simulink model "RL_Model"  (R2025b)
settings: Solver=ode14x  StartTime=0  StopTime=100  FixedStep=simStepSize  RelTol=1e-3
undefined symbols (not defined in the file or in its folder): Defined, driving, Ego, Lane, simStepSize, User
libraries: roadrunnerscenario x6, drivingscenarioandsensors x3, simulink_extras x2, rllib x1
settings Model: Creator=Jacob  LastModifiedBy=balls
settings RTWCC: GPUComputeCapability=3.5

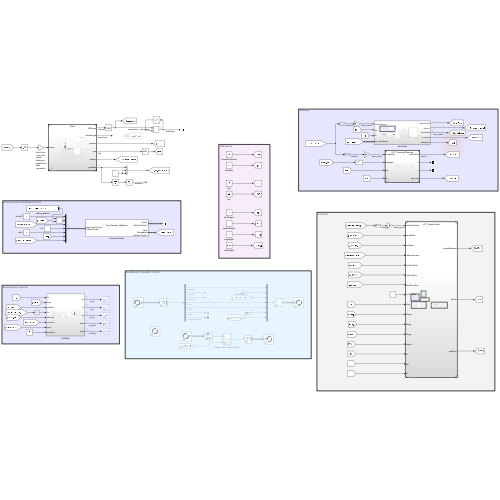
[thumbnail: Simulink's stored preview of the top-level diagram]
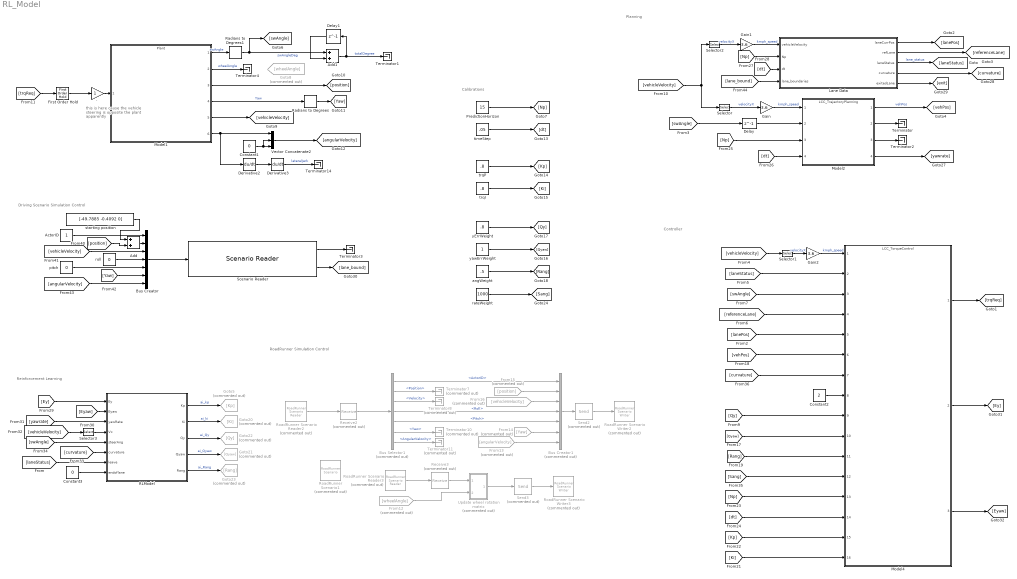
== system RL_Model ==
  note: Driving Scenario Simulation Control
  note: Reinforcement Learning
  note: this is here
      |  cause the
      | vehicle
      | steering is
      | opposite the
      | plant
      |  apparently
  note: Calibrations
  note: Controller
  note: RoadRunner Simulation Control
  note: Planning
  ActorID : Constant
  Add : Sum
  Add1 : Sum
  Bus Creator : BusCreator  Inputs=7  OutDataTypeStr=Bus: BusActorPose  NonVirtualBus=on
      settings: InheritFromInputs=off
  Bus Creator1 : BusCreator  Commented=on  Inputs=7  OutDataTypeStr=Bus: BusActorPose  NonVirtualBus=on
  Bus Selector1 : BusSelector  Commented=on  OutputSignals=ActorID,Position,Velocity,Roll,Pitch,Yaw,AngularVelocity
  Constant1 : Constant  Value=0
  Constant2 : Constant  Value=2
  Constant3 : Constant  Value=0
  Delay : Delay  DelayLength=1
  Delay1 : Delay  DelayLength=1
  Derivative2 : Derivative
  Derivative3 : Derivative
  First Order Hold : FirstOrderHold  ErrorTolerance=inf  AllowContinuousInput=on
  From12 : From  Commented=on  GotoTag=wheelAngle
  From13 : From  Commented=on  GotoTag=angularVelocity
  From14 : From  Commented=on  GotoTag=Yaw
  From15 : From  Commented=on  GotoTag=position
  From16 : From  Commented=on  GotoTag=vehicleVelocity
  Gain : Gain  Gain=3.6
  Gain1 : Gain  Gain=3.6
  Gain2 : Gain  Gain=3.6
  Goto20 : Goto  Commented=on  GotoTag=Ki
  Goto21 : Goto  Commented=on  GotoTag=Qyaw
  Goto22 : Goto  Commented=on  GotoTag=Qy
  Goto23 : Goto  Commented=on  GotoTag=Rang
  Goto5 : Goto  Commented=on  GotoTag=Kp
  Goto8 : Goto  Commented=on  GotoTag=wheelAngle
  Lane Data : Subsystem
  Model1 : ModelReference  ModelNameDialog=Plant.slx  SimulationMode=Normal  ModelReferenceVersion=5.13
  Model2 : ModelReference  ModelNameDialog=LCC_TrajectoryPlanning.slx  SimulationMode=Normal  ModelReferenceVersion=5.4
  Model4 : ModelReference  ModelNameDialog=LCC_TorqueControl.slx  SimulationMode=Normal  ModelReferenceVersion=5.86
  PredictionHorizon : Constant  Value=15
  RLModel : Subsystem
  Radians to Degrees : simulink_extras/Transformations/Radians to Degrees
  Radians to Degrees1 : simulink_extras/Transformations/Radians to Degrees
  Receive2 : Receive  Commented=on  InputPortMessageModes=m  UseInternalQueue=off  QueueOverwriting=on  QueueLength=1  QueueType=LIFO
  Receive3 : Receive  Commented=on  InputPortMessageModes=m  UseInternalQueue=off  QueueOverwriting=on  QueueLength=1  QueueType=LIFO  SampleTime=simStepSize
  RoadRunner Scenario Reader2 : roadrunnerscenario/RoadRunner Scenario Reader  Commented=on  TopicCategory=Actor  ActorCategory=All Types  ActionType=Path Following  EventType=User-Defined  TopicType=Actor Pose (Driving Scenario compatible)  VehicleType=Vehicle Specifications  TrafficSignalType=Traffic Signal Specifications  TrafficSignalControllerType=Traffic Signal Controller Specifications  UserDefinedAction=Action1  UserDefinedEvent=Event1  Filter=Self  AdditionalRelationship=None  SensorTopic=Target Poses  LaneBoundaryOutputTopic=Ego-Lane  SensorID=1  SampleTime=simStepSize
  RoadRunner Scenario Reader3 : roadrunnerscenario/RoadRunner Scenario Reader  Commented=on  TopicCategory=Actor  ActorCategory=Vehicle  ActionType=Path Following  EventType=User-Defined  TopicType=Actor Pose (Driving Scenario compatible)  VehicleType=Vehicle Pose  TrafficSignalType=Traffic Signal Specifications  TrafficSignalControllerType=Traffic Signal Controller Specifications  UserDefinedAction=Action1  UserDefinedEvent=Event1  Filter=Self  AdditionalRelationship=None  SensorTopic=Target Poses  LaneBoundaryOutputTopic=Ego-Lane  SensorID=1  SampleTime=simStepSize
  RoadRunner Scenario Writer2 : roadrunnerscenario/RoadRunner Scenario Writer  Commented=on  TopicCategory=Actor  ActorCategory=All Types  EventType=Action Complete  UserDefinedEvent=Event1  VehicleType=Vehicle Pose  TopicType=Actor Pose (Driving Scenario compatible)
  RoadRunner Scenario Writer3 : roadrunnerscenario/RoadRunner Scenario Writer  Commented=on  TopicCategory=Actor  ActorCategory=Vehicle  EventType=Action Complete  UserDefinedEvent=Event1  VehicleType=Vehicle Pose  TopicType=Actor Pose (Driving Scenario compatible)
  RoadRunner Scenario1 : roadrunnerscenario/RoadRunner Scenario  Commented=on  UserDefinedActions={}  UserDefinedEvents={}  PathPoints=500
  Scenario Reader : drivingscenarioandsensors/Scenario Reader  ScenarioSource=From file  ScenarioFileName=C:\Users\balls\Desktop\EcoCAR\git\CAV - 2025b\Test_Scenario_RightCurv.mat  ScenarioVariableName=scenario  OutputCoordinateSystem=Vehicle coordinates  EgoVehicleSource=Input port  EgoVehicleActorID=1  OrientVehiclesOnRoad=off  OutputEgoVehiclePose=off  OutputEgoVehicleState=off  SampleTime=simStepSize  LaneBoundaryOutput=Ego vehicle lane boundaries  LaneBoundaryDistance=linspace(-150, 150, 101)  LaneBoundaryLocation=Center of lane markings  BusNameSource=Auto  BusName=BusActors  BusNumActorsSource=Scenario  BusNumActors=100  BusName2Source=Auto  BusName2=BusLaneBoundaries  BusNumLaneBoundariesSource=Scenario  BusNumLaneBoundaries=10  BusName3Source=Auto  BusName3=BusEgoActor  BusName4Source=Auto  BusName4=BusEgoState  ShowCoordinateLabels=on  SimulateUsing=Interpreted execution
  Selector{,1..3} (4 alike) : Selector  InputPortWidth=3  IndexOptions=Index vector (dialog)  Indices=1  OutputSizes=1
  Send2 : Send  Commented=on  OutputPortMessageModes=m
  Send3 : Send  Commented=on  OutputPortMessageModes=m
  Terminator{,1..4,14} (6 alike) : Terminator
  Terminator{7..8,10..11} (4 alike) : Terminator  Commented=on
  Update wheel rotation matrix : Subsystem  Commented=on
  Vector Concatenate2 : Concatenate  NumInputs=3  Mode=Multidimensional array  ConcatenateDimension=2
  ` : Gain
  angWeight : Constant  Value=.5
  pitch : Constant  Value=0
  rateWeight : Constant  Value=1000
  roll : Constant  Value=0
  starting position : Constant  Value=[-49.7885 -0.4092 0]
  timeStep : Constant  Value=.05
  trqI : Constant  Value=.8
  trqP : Constant  Value=.8
  yErrWeight : Constant  Value=.8
  yawErrWeight : Constant
  wires:
  Delay1/1 -> Add1/2
  Radians to Degrees1/1 -> [swAngle], Add1/1  "swAngleDeg"
  Bus Selector1/4 -> Bus Creator1/4  "<Roll>"
  From14/1 -> Bus Creator1/6
  Add1/1 -> Terminator1/1, Delay1/1  "totalDegree"
  Bus Selector1/2 -> Terminator7/1  "<Position>"
  Bus Selector1/7 -> Terminator11/1  "<AngularVelocity>"
  Model1/3 -> [position]
  Bus Selector1/1 -> Bus Creator1/1  "<ActorID>"
  RoadRunner Scenario Reader3/1 -> Receive3/1
  Send3/1 -> RoadRunner Scenario Writer3/1
  From15/1 -> Bus Creator1/2
  Model1/4 -> Radians to Degrees/1  "Yaw"
  Derivative2/1 -> Derivative3/1
  Send2/1 -> RoadRunner Scenario Writer2/1
  Model1/1 -> Radians to Degrees1/1  "swAngle"
  Bus Creator1/1 -> Send2/1
  RoadRunner Scenario Reader2/1 -> Receive2/1
  Radians to Degrees/1 -> [Yaw]
  Bus Selector1/5 -> Bus Creator1/5  "<Pitch>"
  Model2/1 -> [vehPos]  "vehPos"
  Receive2/1 -> Bus Selector1/1
  [vehicleVelocity] -> Selector2/1, Selector/1
  Vector Concatenate2/1 -> [angularVelocity]
  Bus Selector1/6 -> Terminator10/1  "<Yaw>"
  Constant1/1 -> Vector Concatenate2/2, Vector Concatenate2/3
  From16/1 -> Bus Creator1/3
  Derivative3/1 -> Terminator14/1  "lateralJerk"
  From13/1 -> Bus Creator1/7
  Model1/5 -> [vehicleVelocity]
  Bus Selector1/3 -> Terminator8/1  "<Velocity>"
  [trqReq] -> First Order Hold/1
  Lane Data/3(laneStatus) -> [laneStatus]  "lane_status"
  Model1/6 -> Derivative2/1, Vector Concatenate2/1
  Selector/1 -> Gain/1  "velocityX"
  Gain/1 -> Model2/1  "kmph_speed"
  Delay/1 -> Model2/2
  First Order Hold/1 -> `/1
  Lane Data/1(laneCurrPos) -> [lanePos]
  [vehicleVelocity] -> Selector1/1
  Selector1/1 -> Gain2/1  "velocityX"
  [swAngle] -> Delay/1
  Receive3/1 -> Update wheel rotation matrix/1(In1)
  Update wheel rotation matrix/1(Out1) -> Send3/1
  From12/1 -> Update wheel rotation matrix/2(Input)
  [vehPos] -> Model4/6
  [Np] -> Model2/3
  [dt] -> Model2/4
  angWeight/1 -> [Rang]
  yawErrWeight/1 -> [Qyaw]
  yErrWeight/1 -> [Qy]
  trqI/1 -> [Ki]
  trqP/1 -> [Kp]
  timeStep/1 -> [dt]
  PredictionHorizon/1 -> [Np]
  [Qy] -> Model4/9
  [Qyaw] -> Model4/10
  [Rang] -> Model4/11
  [Np] -> Model4/13
  [dt] -> Model4/14
  [Np] -> Lane Data/2(Np)
  [dt] -> Lane Data/3(dt)
  Model4/1 -> [trqReq]
  Selector2/1 -> Gain1/1  "velocityX"
  Gain1/1 -> Lane Data/1(vehicleVelocity)  "kmph_speed"
  Lane Data/2(refLane) -> [referenceLane]
  `/1 -> Model1/1
  RLModel/1(Kp) -> Goto5/1  "ai_kp"
  RLModel/2(Ki) -> Goto20/1  "ai_ki"
  RLModel/3(Qy) -> Goto22/1  "ai_Qy"
  RLModel/4(Qyaw) -> Goto21/1  "ai_Qyaw"
  RLModel/5(Rang) -> Goto23/1  "ai_Rang"
  [Ey] -> RLModel/1(Ey)
  [Eyaw] -> RLModel/2(Eyaw)
  [yawrate] -> RLModel/3(yawRate)
  [vehicleVelocity] -> Selector3/1
  Lane Data/4(curvature) -> [curvature]
  [curvature] -> RLModel/6(curvature)
  [swAngle] -> RLModel/5(steerAng)
  rateWeight/1 -> [Sang]
  [Sang] -> Model4/12
  [curvature] -> Model4/7
  Constant2/1 -> Model4/8
  Lane Data/5(exitedLane) -> [exit]
  [laneStatus] -> RLModel/7(leave)
  Model2/4 -> [yawrate]
  Model2/2 -> Terminator/1
  Model2/3 -> Terminator2/1
  Constant3/1 -> RLModel/8(endoflane)
  Selector3/1 -> RLModel/4(Vx)
  Scenario Reader/2 -> [lane_bound]
  Scenario Reader/1 -> Terminator3/1
  [lane_bound] -> Lane Data/4(lane_boundaries)
  Model1/2 -> Terminator4/1  "wheelAngle"
  ActorID/1 -> Bus Creator/1
  [angularVelocity] -> Bus Creator/7
  [vehicleVelocity] -> Bus Creator/3
  pitch/1 -> Bus Creator/5
  roll/1 -> Bus Creator/4
  [Yaw] -> Bus Creator/6
  Bus Creator/1 -> Scenario Reader/1
  [position] -> Add/2
  starting position/1 -> Add/1
  Add/1 -> Bus Creator/2
  [Kp] -> Model4/15
  [Ki] -> Model4/16
  [lanePos] -> Model4/5
  [referenceLane] -> Model4/4
  Gain2/1 -> Model4/1  "kmph_speed"
  [swAngle] -> Model4/3
  [laneStatus] -> Model4/2
  Model4/2 -> [Ey]
  Model4/3 -> [Eyaw]

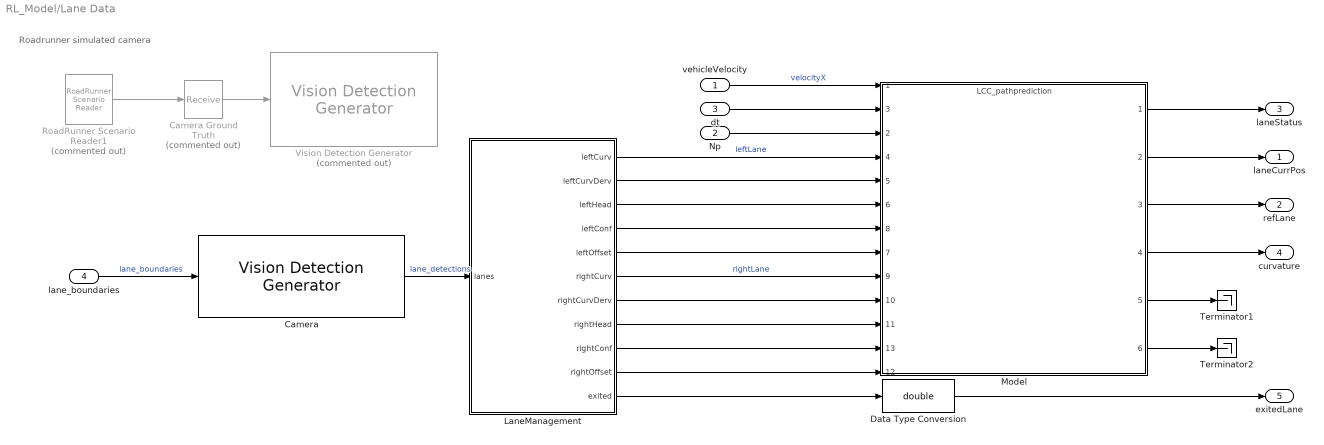
== system RL_Model/Lane Data ==
  note: Roadrunner simulated camera
  vehicleVelocity : Inport
  Np : Inport  Port=2
  dt : Inport  Port=3
  lane_boundaries : Inport  Port=4
  Camera : drivingscenarioandsensors/Vision Detection Generator  SensorIndex=1  DetectorOutput=Lanes only  UpdateInterval=0.1  LaneUpdateInterval=0.1  SensorLocation=[1.9 0]  Height=1.1  Yaw=0  Pitch=1  Roll=0  BusNameSource=Auto  BusName=BusObjectDetections  BusName2Source=Auto  BusName2=BusLaneDetections  MaxNumDetectionsSource=Property  MaxNumDetections=50  MaxNumLanesSource=Property  MaxNumLanes=30  DetectionCoordinates=Ego Cartesian  SimulateUsing=Interpreted execution  MaxRange=150  BoundingBoxAccuracy=5  ProcessNoiseIntensity=5  MaxSpeed=100  MaxAllowedOcclusion=0.5  MinObjectImageSize=[15 15]  DetectionProbability=0.9  FalsePositivesPerImage=0.1  MinLaneImageSize=[20 3]  LaneBoundaryAccuracy=3  HasNoise=on  InitialSeedSource=Repeatable  InitialSeed=0  UsedSeed=0  ActorProfilesSource=From Scenario Reader block  ActorProfilesParameters=driving.internal.ActorProfilesParameters  ActorProfilesExpression=[struct('ActorID',1,'ClassID',1,'Length',4.7,'Width',1.8,'Height',1.4,'OriginOffset',[-1.35 0 0],'MeshVertices',[3.7 0.9 0.857439446366782;3.7 -0.9 0.857439446366782;3.7 -0.9 0.314878892733564;3.7 0.9 0.314878892733564;3.7 0.9 0.857439446366782;2.525 0.9 0.993079584775086;2.525 -0.9 0.993079584775086;3.7 -0.9 0.857439446366782;1.82 0.72 1.4;0.41 0.72 1.4;0.41 -0.72 1.4;1.82 -0.72 1.4;-0.295 0.9 0.993079584775086;-1 0.9 0.857439446366782;-1 -0.9 0.857439446366782;-0.295 -0.9 0.993079584775086;3.7 0.9 0.857439446366782;3.7 0.9 0.314878892733564;2.525 0.9 0.314878892733564;2.525 0.9 0.993079584775086;2.525 0.9 0.993079584775086;2.525 0.9 0.314878892733564;-0.295 0.9 0.314878892733564;-0.295 0.9 0.993079584775086;-0.295 0.9 0.993079584775086;-0.295 0.9 0.314878892733564;-1 0.9 0.355570934256055;-1 0.9 0.857439446366782;2.525 0.9 0.993079584775086;-0.295 0.9 0.993079584775086;0.41 0.72 1.4;1.82 0.72 1.4;3.7 -0.9 0.857439446366782;3.7 -0.9 0.314878892733564;2.525 -0.9 0.314878892733564;2.525 -0.9 0.993079584775086;2.525 -0.9 0.993079584775086;2.525 -0.9 0.314878892733564;-0.295 -0.9 0.314878892733564;-0.295 -0.9 0.993079584775086;-0.295 -0.9 0.993079584775086;-0.295 -0.9 0.314878892733564;-1 -0.9 0.355570934256055;-1 -0.9 0.857439446366782;2.525 -0.9 0.993079584775086;-0.295 -0.9 0.993079584775086;0.41 -0.72 1.4;1.82 -0.72 1.4;-0.295 0.9 0.993079584775086;-0.295 -0.9 0.993079584775086;0.41 -0.72 1.4;0.41 0.72 1.4;2.525 -0.9 0.993079584775086;1.82 -0.72 1.4;1.82 0.72 1.4;2.525 0.9 0.993079584775086;-1 0.9 0.857439446366782;-1 0.9 0.355570934256055;-1 -0.9 0.355570934256055;-1 -0.9 0.857439446366782;3.7 0.9 0.314878892733564;3.7 -0.9 0.314878892733564;-0.295 -0.9 0.314878892733564;-0.295 0.9 0.314878892733564;-0.295 0.9 0.314878892733564;-1 0.9 0.355570934256055;-1 -0.9 0.355570934256055;-0.295 -0.9 0.314878892733564;0 -0.63 0;0 -0.87 0;0.191030206995054 -0.63 0.0601365173421445;0.191030206995054 -0.87 0.0601365173421445;0.309093367795925 -0.63 0.217575963708927;0.309093367795925 -0.87 0.217575963708927;0.309093367795925 -0.63 0.412181821758201;0.309093367795925 -0.87 0.412181821758201;0.191030206995054 -0.63 0.569621268124983;0.191030206995054 -0.87 0.569621268124983;0 -0.63 0.629757785467128;0 -0.87 0.629757785467128;-0.191030206995054 -0.63 0.569621268124983;-0.191030206995054 -0.87 0.569621268124983;-0.309093367795925 -0.63 0.412181821758201;-0.309093367795925 -0.87 0.412181821758201;-0.309093367795925 -0.63 0.217575963708927;-0.309093367795925 -0.87 0.217575963708927;-0.191030206995054 -0.63 0.0601365173421445;-0.191030206995054 -0.87 0.0601365173421445;0 -0.63 0;0 -0.87 0;0 -0.63 0;0.191030206995054 -0.63 0.0601365173421445;0.309093367795925 -0.63 0.217575963708927;0.309093367795925 -0.63 0.412181821758201;0.191030206995054 -0.63 0.569621268124983;0 -0.63 0.629757785467128;-0.191030206995054 -0.63 0.569621268124983;-0.309093367795925 -0.63 0.412181821758201;-0.309093367795925 -0.63 0.217575963708927;-0.191030206995054 -0.63 0.0601365173421445;0 -0.87 0;0.191030206995054 -0.87 0.0601365173421445;0.309093367795925 -0.87 0.217575963708927;0.309093367795925 -0.87 0.412181821758201;0.191030206995054 -0.87 0.569621268124983;0 -0.87 0.629757785467128;-0.191030206995054 -0.87 0.569621268124983;-0.309093367795925 -0.87 0.412181821758201;-0.309093367795925 -0.87 0.217575963708927;-0.191030206995054 -0.87 0.0601365173421445;0 0.87 0;0 0.63 0;0.191030206995054 0.87 0.0601365173421445;0.191030206995054 0.63 0.0601365173421445;0.309093367795925 0.87 0.217575963708927;0.309093367795925 0.63 0.217575963708927;0.309093367795925 0.87 0.412181821758201;0.309093367795925 0.63 0.412181821758201;0.191030206995054 0.87 0.569621268124983;0.191030206995054 0.63 0.569621268124983;0 0.87 0.629757785467128;0 0.63 0.629757785467128;-0.191030206995054 0.87 0.569621268124983;-0.191030206995054 0.63 0.569621268124983;-0.309093367795925 0.87 0.412181821758201;-0.309093367795925 0.63 0.412181821758201;-0.309093367795925 0.87 0.217575963708927;-0.309093367795925 0.63 0.217575963708927;-0.191030206995054 0.87 0.0601365173421445;-0.191030206995054 0.63 0.0601365173421445;0 ...(+3718 chars)],'MeshFaces',[1 2 3;3 4 1;5 6 7;7 8 5;9 10 11;11 12 9;13 14 15;15 16 13;17 18 19;19 20 17;21 22 23;23 24 21;25 26 27;27 28 25;29 30 31;31 32 29;33 34 35;35 36 33;37 38 39;39 40 37;41 42 43;43 44 41;45 46 47;47 48 45;49 50 51;51 52 49;53 54 55;55 56 53;57 58 59;59 60 57;61 62 63;63 64 61;65 66 67;67 68 65;69 71 72;72 70 69;71 73 74;74 72 71;73 75 76;76 74 73;75 77 78;78 76 75;77 79 80;80 78 77;79 81 82;82 80 79;81 83 84;84 82 81;83 85 86;86 84 83;85 87 88;88 86 85;87 89 90;90 88 87;91 92 93;91 93 94;91 94 95;91 95 96;91 96 97;91 97 98;91 98 99;91 99 100;101 102 103;101 103 104;101 104 105;101 105 106;101 106 107;101 107 108;101 108 109;101 109 110;111 113 114;114 112 111;113 115 116;116 114 113;115 117 118;118 116 115;117 119 120;120 118 117;119 121 122;122 120 119;121 123 124;124 122 121;123 125 126;126 124 123;125 127 128;128 126 125;127 129 130;130 128 127;129 131 132;132 130 129;133 134 135;133 135 136;133 136 137;133 137 138;133 138 139;133 139 140;133 140 141;133 141 142;143 144 145;143 145 146;143 146 147;143 147 148;143 148 149;143 149 150;143 150 151;143 151 152;153 155 156;156 154 153;155 157 158;158 156 155;157 159 160;160 158 157;159 161 162;162 160 159;161 163 164;164 162 161;163 165 166;166 164 163;165 167 168;168 166 165;167 169 170;170 168 167;169 171 172;172 170 169;171 173 174;174 172 171;175 176 177;175 177 178;175 178 179;175 179 180;175 180 181;175 181 182;175 182 183;175 183 184;185 186 187;185 187 188;185 188 189;185 189 190;185 190 191;185 191 192;185 192 193;185 193 194;195 197 198;198 196 195;197 199 200;200 198 197;199 201 202;202 200 199;201 203 204;204 202 201;203 205 206;206 204 203;205 207 208;208 206 205;207 209 210;210 208 207;209 211 212;212 210 209;211 213 214;214 212 211;213 215 216;216 214 213;217 218 219;217 219 220;217 220 221;217 221 222;217 222 223;217 223 224;217 224 225;217 225 226;227 228 229;227 229 230;227 230 231;227 231 232;227 232 233;227 233 234;227 234 235;227 235 236],'RCSPattern',[10 10;10 10],'RCSAzimuthAngles',[-180 180],'RCSElevationAngles',[-90 90])]  Intrinsics=driving.internal.cameraIntrinsics('FocalLength',[800 800],'PrincipalPoint',[320 240],'ImageSize',[480 640],'RadialDistortion',[0 0],'TangentialDistortion',[0 0],'Skew',0)
  Camera Ground Truth : Receive  Commented=on  InputPortMessageModes=m  UseInternalQueue=off  QueueOverwriting=on  QueueLength=1  QueueType=LIFO  SampleTime=simStepSize
  Data Type Conversion : DataTypeConversion  OutDataTypeStr=double  SaturateOnIntegerOverflow=off  RndMeth=Floor
  LaneManagement : MATLAB Function  TreatAsAtomicUnit=on
  Model : ModelReference  ModelNameDialog=LCC_pathprediction.slx  SimulationMode=Normal  ModelReferenceVersion=5.49
      settings: PortSchema="{\"entries\":[{\"content\":{\"sides\":[{\"content\":{\"connectorIds\":[\"In1\",\"In3\",\"In2\",\"In4\",\"In5\",\"In6\",\"In8\",\"In7\",\"In9\",\"In10\",\"In11\",\"In13\",\"In12\"]},\"type\":\"ConnectorPlacement.EquallySpacedRectSide\",\"uuid\":\"a07f8485-8c73-44ce-93cf-ec5e6f63c5da\"},{\"content\":{\"connectorIds\":[\"Out1\",\"Out2\",\"Out3\",\"Out4\",\"Out5\",\"Out6\"],\"side\":\"RIGHT\"},\"type\":\"ConnectorPlacement.EquallySpacedRectSide\",\"uuid\":\"b69156b0-73a0-4176-8c64-fda440ac3685\"},{\"content\":{\"side\":\"TOP\"},\"type\":\"ConnectorPlacement.EquallySpacedRectSide\",\"uuid\":\"33404bc1-182d-48ae-8070-d21d23a4a197\"}]},\"type\":\"ConnectorPlacement.EquallySpacedConnector\",\"uuid\":\"de203df0-0780-4dcc-b040-a4939f0923fa\"}],\"packageUris\":[\"http://schema.mathworks.com/mf0/Connector/R2020b\"],\"version\":\"1.0\"}"
  RoadRunner Scenario Reader1 : roadrunnerscenario/RoadRunner Scenario Reader  Commented=on  TopicCategory=Sensor  ActorCategory=All Types  ActionType=Path Following  EventType=User-Defined  TopicType=Actor Specifications  VehicleType=Vehicle Specifications  TrafficSignalType=Traffic Signal Specifications  TrafficSignalControllerType=Traffic Signal Controller Specifications  UserDefinedAction=Action1  UserDefinedEvent=Event1  Filter=Self  AdditionalRelationship=None  SensorTopic=Lane Boundaries  LaneBoundaryOutputTopic=Ego and Adjacent Lanes  SensorID=1  SampleTime=simStepSize
  Terminator1 : Terminator
  Terminator2 : Terminator
  Vision Detection Generator : drivingscenarioandsensors/Vision Detection Generator  Commented=on  SensorIndex=1  DetectorOutput=Lanes only  UpdateInterval=simStepSize  LaneUpdateInterval=simStepSize  SensorLocation=[ 1, 0 ]  Height=1.9  Yaw=0  Pitch=1  Roll=0  BusNameSource=Auto  BusName=BusObjectDetections  BusName2Source=Auto  BusName2=BusLaneDetections  MaxNumDetectionsSource=Property  MaxNumDetections=10  MaxNumLanesSource=Property  MaxNumLanes=10  DetectionCoordinates=Ego Cartesian  SimulateUsing=Code generation  MaxRange=100  BoundingBoxAccuracy=5  ProcessNoiseIntensity=5  MaxSpeed=100  MaxAllowedOcclusion=0.5  MinObjectImageSize=[ 5, 5 ]  DetectionProbability=0.99  FalsePositivesPerImage=0.01  MinLaneImageSize=[ 20, 3 ]  LaneBoundaryAccuracy=3  HasNoise=on  InitialSeedSource=Repeatable  InitialSeed=0  UsedSeed=driving.internal.SimulinkUtilities.seedManager(gcb)  ActorProfilesSource=From Scenario Reader block  ActorProfilesParameters=driving.internal.ActorProfilesParameters  ActorProfilesExpression=struct( 'ClassID', 0, 'Length', 4.7, 'Width', 1.8, 'Height', 1.4, 'OriginOffset', [ -1.35, 0, 0 ] )  Intrinsics=driving.internal.cameraIntrinsics
  laneCurrPos : Outport
  refLane : Outport  Port=2
  laneStatus : Outport  Port=3
  curvature : Outport  Port=4
  exitedLane : Outport  Port=5
  wires:
  RoadRunner Scenario Reader1/1 -> Camera Ground Truth/1
  Model/1 -> laneStatus/1
  Model/2 -> laneCurrPos/1
  Model/3 -> refLane/1
  vehicleVelocity/1 -> Model/1  "velocityX"
  Np/1 -> Model/2
  dt/1 -> Model/3
  Model/5 -> Terminator1/1
  Model/4 -> curvature/1
  LaneManagement/1(leftCurv) -> Model/4  "leftLane"
  LaneManagement/2(leftCurvDerv) -> Model/5
  LaneManagement/3(leftHead) -> Model/6
  LaneManagement/4(leftConf) -> Model/8
  LaneManagement/5(leftOffset) -> Model/7
  LaneManagement/6(rightCurv) -> Model/9  "rightLane"
  LaneManagement/10(rightOffset) -> Model/12
  LaneManagement/9(rightConf) -> Model/13
  LaneManagement/8(rightHead) -> Model/11
  LaneManagement/7(rightCurvDerv) -> Model/10
  Data Type Conversion/1 -> exitedLane/1
  LaneManagement/11(exited) -> Data Type Conversion/1
  Camera Ground Truth/1 -> Vision Detection Generator/1
  Camera/1 -> LaneManagement/1(lanes)  "lane_detections"
  lane_boundaries/1 -> Camera/1  "lane_boundaries"
  Model/6 -> Terminator2/1

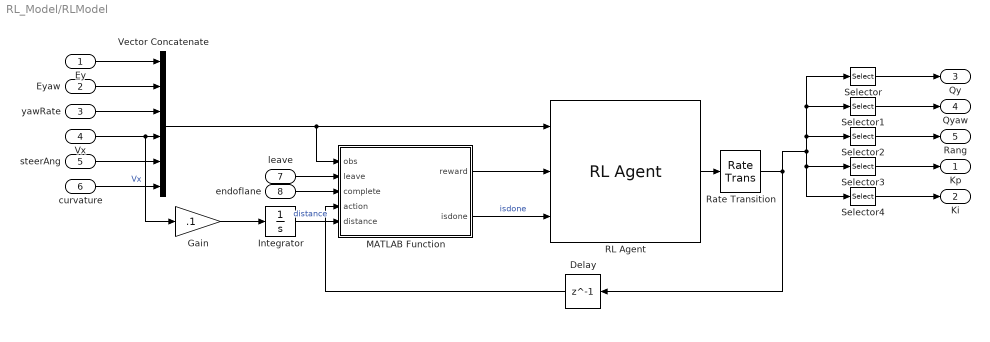
== system RL_Model/RLModel ==
  Ey : Inport
  Eyaw : Inport  Port=2
  yawRate : Inport  Port=3
  Vx : Inport  Port=4
  steerAng : Inport  Port=5
  curvature : Inport  Port=6
  leave : Inport  Port=7
  endoflane : Inport  Port=8
  Delay : Delay  DelayLength=1
  Gain : Gain  Gain=.1
  Integrator : Integrator
  MATLAB Function : MATLAB Function  TreatAsAtomicUnit=on
  RL Agent : rllib/RL Agent  Agent=agent_Trained  ExternalActionAsInput=off  ProvideLastAction=off  ProvideCumRwd=off  TreatAsDirectFeedthrough=on  UseStrictObservationDataTypes=off
  Rate Transition : RateTransition  OutPortSampleTime=simStepSize
  Selector : Selector  InputPortWidth=5  IndexOptions=Index vector (dialog)  Indices=1  OutputSizes=1
  Selector1 : Selector  InputPortWidth=5  IndexOptions=Index vector (dialog)  Indices=2  OutputSizes=1
  Selector2 : Selector  InputPortWidth=5  IndexOptions=Index vector (dialog)  Indices=3  OutputSizes=1
  Selector3 : Selector  InputPortWidth=5  IndexOptions=Index vector (dialog)  Indices=4  OutputSizes=1
  Selector4 : Selector  InputPortWidth=5  IndexOptions=Index vector (dialog)  Indices=5  OutputSizes=1
  Vector Concatenate : Concatenate  NumInputs=6  Mode=Multidimensional array
  Kp : Outport
  Ki : Outport  Port=2
  Qy : Outport  Port=3
  Qyaw : Outport  Port=4
  Rang : Outport  Port=5
  wires:
  Vector Concatenate/1 -> RL Agent/1, MATLAB Function/1(obs)
  steerAng/1 -> Vector Concatenate/5
  RL Agent/1 -> Rate Transition/1
  curvature/1 -> Vector Concatenate/6
  yawRate/1 -> Vector Concatenate/3
  Vx/1 -> Gain/1, Vector Concatenate/4  "Vx"
  Ey/1 -> Vector Concatenate/1
  Eyaw/1 -> Vector Concatenate/2
  Selector3/1 -> Kp/1
  Selector2/1 -> Rang/1
  Selector1/1 -> Qyaw/1
  Selector/1 -> Qy/1
  Selector4/1 -> Ki/1
  MATLAB Function/1(reward) -> RL Agent/2
  endoflane/1 -> MATLAB Function/3(complete)
  leave/1 -> MATLAB Function/2(leave)
  Delay/1 -> MATLAB Function/4(action)
  Rate Transition/1 -> Delay/1, Selector/1, Selector1/1, Selector2/1, Selector4/1, Selector3/1
  MATLAB Function/2(isdone) -> RL Agent/3  "isdone"
  Integrator/1 -> MATLAB Function/5(distance)  "distance"
  Gain/1 -> Integrator/1

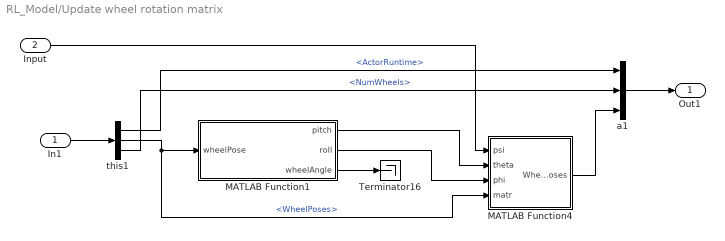
== system RL_Model/Update wheel rotation matrix ==
  In1 : Inport
  Input : Inport  Port=2
  MATLAB Function1 : MATLAB Function  TreatAsAtomicUnit=on
  MATLAB Function4 : MATLAB Function  TreatAsAtomicUnit=on
  Terminator16 : Terminator
  a1 : BusCreator  Inputs=3  OutDataTypeStr=Bus: BusVehicleRuntime  NonVirtualBus=on
  this1 : BusSelector  OutputSignals=ActorRuntime,WheelPoses,NumWheels
  Out1 : Outport
  wires:
  MATLAB Function1/1(pitch) -> MATLAB Function4/2(theta)
  this1/2 -> MATLAB Function4/4(matr), MATLAB Function1/1(wheelPose)  "<WheelPoses>"
  In1/1 -> this1/1
  MATLAB Function1/2(roll) -> MATLAB Function4/3(phi)
  this1/1 -> a1/1  "<ActorRuntime>"
  this1/3 -> a1/2  "<NumWheels>"
  MATLAB Function4/1(WheelPoses) -> a1/3
  MATLAB Function1/3(wheelAngle) -> Terminator16/1
  a1/1 -> Out1/1
  Input/1 -> MATLAB Function4/1(psi)

== matlab function RL_Model/RLModel/MATLAB Function ==
  settings: updateMethod=DISCRETE
  data: obs input double size=[6, 1]; reward output double size=1; leave input double size=1; complete input double size=1; action input double size=[5, 1]; isdone output boolean size=1; distance input
    function [reward, isdone] = fcn(obs, leave, complete, action, distance)

persistent steer_prev

if isempty(leave)
    left = 0;
else
    left = leave;
end

if isempty(complete)
    done = 0;
else
    done = complete;
end

isdone = ~left || done;

%% Reward Function
% Reward Function Weights
cy = .25;
cyaw = .1;
crate = 1;

offy = .005;
offyaw = .005;
offrate = 0;

if isempty(obs)
    obs = zeros(6);
end
% more error, bad. Each error
Ey = obs(1);
Eyaw = obs(2);

% More yaw rate, bad? this will lead to higher jerk
yawRate = obs(3);

% compare lane curvature K to vehicle curvature
Vx = obs(4);
if Vx == 0
    Vx = .01;
end

k_veh = yawRate/ Vx;
    
k_lane = obs(6);
    
k_diff = k_lane - k_veh;
    
% penalize steering angle change
steerAng = obs(5);
    
if isempty(steer_prev)
    steer_prev = steerAng;
end
    
steer_dot = steerAng - steer_prev;
steer_prev = steerAng;

reward = (-cy*Ey^2 + offy) + (-cyaw*Eyaw^2 + offyaw) + (-crate*yawRate + offrate) - k_diff - steer_dot + 5*done - 5*left + distance;

== matlab function RL_Model/Lane Data/LaneManagement ==
  data: lanes input size=[1 1]; leftCurv output; leftCurvDerv output; leftHead output; leftConf output; leftOffset output; rightCurv output; rightCurvDerv output; rightHead output; rightConf output; rightOffset output; exited output
function [leftCurv, leftCurvDerv, leftHead, leftConf, leftOffset, rightCurv, rightCurvDerv, rightHead, rightConf, rightOffset, exited] = LaneManagement(lanes)

leftCurv = 0;
leftCurvDerv = 0;
leftHead = 0;
leftConf = 0;
leftOffset = 0;

rightCurv = 0;
rightCurvDerv = 0;
rightHead = 0;
rightConf = 0;
rightOffset = 0;

exited = 0;

for i=1:lanes.NumLaneBoundaries
    
    if (lanes.LaneBoundaries(i).LateralOffset > 0) && (lanes.LaneBoundaries(i).LateralOffset < 5)
        leftCurv = double(lanes.LaneBoundaries(i).Curvature);
        leftCurvDerv = double(lanes.LaneBoundaries(i).CurvatureDerivative);
        leftHead = double(lanes.LaneBoundaries(i).HeadingAngle);
        leftOffset = double(lanes.LaneBoundaries(i).LateralOffset);
        leftConf = double(1);

    elseif (lanes.LaneBoundaries(i).LateralOffset < 0) && (lanes.LaneBoundaries(i).LateralOffset > -5)
        rightCurv = double(lanes.LaneBoundaries(i).Curvature);
        rightCurvDerv = double(lanes.LaneBoundaries(i).CurvatureDerivative);
        rightHead = double(lanes.LaneBoundaries(i).HeadingAngle);
        rightOffset = double(lanes.LaneBoundaries(i).LateralOffset);
        rightConf = double(1);
    end


    if (leftCurv == 0) & (rightCurv == 0)
        exited = 1;
    end

end

== matlab function RL_Model/Update wheel rotation matrix/MATLAB Function1 ==
  data: pitch output; roll output; wheelPose input; wheelAngle output
function [pitch, roll, wheelAngle] = wheelPoseTOwheelAngle(wheelPose)
    
    rotation = wheelPose(1:3, 1:3);
    eul = rotm2eul(rotation, "ZYX");
    pitch = eul(3);
    roll = eul(2);
    wheelAngle = eul(1);

end

== matlab function RL_Model/Update wheel rotation matrix/MATLAB Function4 ==
  data: psi input; WheelPoses output; theta input; phi input; matr input
function WheelPoses = fcn(psi, theta, phi, matr)
% psi-yaw  theta-pitch  phi-roll
rotation = [cos(psi)*cos(theta)   sin(psi)*cos(theta)   -sin(theta);
        cos(psi)*sin(theta)*sin(phi)   sin(psi)*sin(theta)*sin(phi)+cos(psi)*cos(phi)   cos(theta)*sin(phi); 
        cos(psi)*sin(theta)*cos(phi)+sin(psi)*sin(theta)   sin(psi)*sin(theta)*cos(phi)-cos(psi)*sin(phi)   cos(theta)*cos(phi)];

matr(1:3, 1:3) = rotation;
WheelPoses = matr;
end
